simulink model "all_phase"  (Simulink 10.0)
settings: Solver=ode45  StartTime=0.0  StopTime=10.0  RelTol=1e-3  EnableMultiTasking=on
settings Model: Creator=bhisma  LastModifiedBy=bhisma
settings DataIOCC: LimitDataPoints=on  SignalLoggingSaveFormat=ModelDataLogs  SignalLoggingName=sigsOut
settings OptimizationCC: BlockReduction=off  BooleanDataType=off  LifeSpan=auto
settings DebuggingCC: SaveWithParameterizedLinksMsg=none  SignalResolutionControl=TryResolveAllWithWarning  MultiTaskDSMMsg=warning  MultiTaskCondExecSysMsg=none  SFUnexpectedBacktrackingDiag=error  SFNoUnconditionalDefaultTransitionDiag=error  SFExecutionAtInitializationDiag=warning  ArithmeticOperatorsInVariantConditions=error
settings HardwareCC: TargetUnknown=on
settings SFSimCC: SimUseLocalCustomCode=on  CustomCodeUndefinedFunction=FilterOut
settings RTWCC: RTWUseLocalCustomCode=on
settings CodeAppCC: StateflowObjectComments=off
settings GRTTargetCC: TargetLangStandard=C99 (ISO)

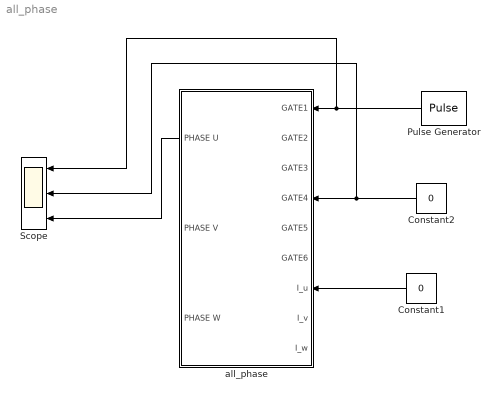
== system all_phase ==
  Constant1 : Constant  Value=0
  Constant2 : Constant  Value=0
  Pulse Generator : DiscretePulseGenerator  PulseType=Time based  Amplitude=100  Period=0.2  PulseWidth=50
  Scope : Scope  NumInputPorts=3
  all_phase : Subsystem  mask{BV=160}
      mask prompts: BV "Battery voltage for excitation"
      mask help: This is an inverter. Double click the block to enter the battery voltage
  wires:
  Pulse Generator/1 -> all_phase/1(GATE1), Scope/1
  Constant2/1 -> all_phase/4(GATE4), Scope/2
  Constant1/1 -> all_phase/7(I_u)
  all_phase/1(PHASE U) -> Scope/3

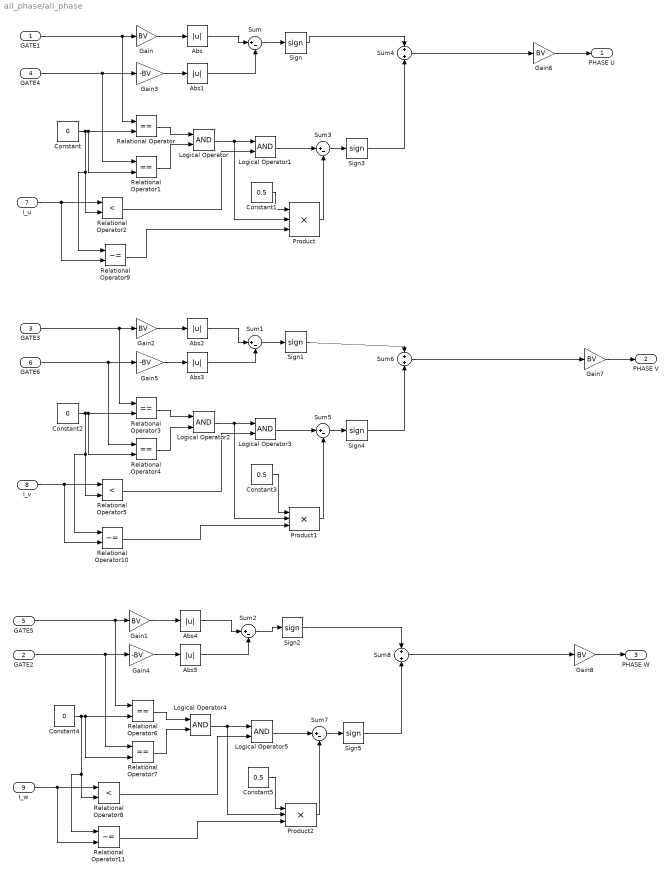
== system all_phase/all_phase ==
  GATE1 : Inport
  GATE2 : Inport  Port=2
  GATE3 : Inport  Port=3
  GATE4 : Inport  Port=4
  GATE5 : Inport  Port=5
  GATE6 : Inport  Port=6
  I_u : Inport  Port=7
  I_v : Inport  Port=8
  I_w : Inport  Port=9
  Abs{,1..5} (6 alike) : Abs  SaturateOnIntegerOverflow=on
  Constant : Constant  Value=0
  Constant1 : Constant  Value=0.5
  Constant2 : Constant  Value=0
  Constant3 : Constant  Value=0.5
  Constant4 : Constant  Value=0
  Constant5 : Constant  Value=0.5
  Gain{,1..2,6..8} (6 alike) : Gain  Gain=BV  SaturateOnIntegerOverflow=on  OutDataTypeStr=Inherit: Same as input  ParamDataTypeStr=Inherit: Same as input
  Gain3 : Gain  Gain=-BV  SaturateOnIntegerOverflow=on  OutDataTypeStr=Inherit: Same as input  ParamDataTypeStr=Inherit: Same as input
  Gain4 : Gain  Gain=-BV  SaturateOnIntegerOverflow=on  OutDataTypeStr=Inherit: Same as input  ParamDataTypeStr=Inherit: Same as input
  Gain5 : Gain  Gain=-BV  SaturateOnIntegerOverflow=on  OutDataTypeStr=Inherit: Same as input  ParamDataTypeStr=Inherit: Same as input
  Logical Operator{,1..5} (6 alike) : Logic  AllPortsSameDT=off
  Product : Product  Inputs=3  SaturateOnIntegerOverflow=on  OutDataTypeStr=Inherit: Same as first input
  Product1 : Product  Inputs=3  SaturateOnIntegerOverflow=on  OutDataTypeStr=Inherit: Same as first input
  Product2 : Product  Inputs=3  SaturateOnIntegerOverflow=on  OutDataTypeStr=Inherit: Same as first input
  Relational Operator{,1,3..4,6..7} (6 alike) : RelationalOperator  Operator===  RndMeth=Nearest
  Relational Operator10 : RelationalOperator  Operator=~=  RndMeth=Nearest
  Relational Operator11 : RelationalOperator  Operator=~=  RndMeth=Nearest
  Relational Operator2 : RelationalOperator  Operator=<  RndMeth=Nearest
  Relational Operator5 : RelationalOperator  Operator=<  RndMeth=Nearest
  Relational Operator8 : RelationalOperator  Operator=<  RndMeth=Nearest
  Relational Operator9 : RelationalOperator  Operator=~=  RndMeth=Nearest
  Sign{,1..5} (6 alike) : Signum
  Sum{,1..3,5,7} (6 alike) : Sum  Inputs=|+-  SaturateOnIntegerOverflow=on  InputSameDT=on  OutDataTypeStr=Inherit: Same as first input
  Sum4 : Sum  SaturateOnIntegerOverflow=on  InputSameDT=on  OutDataTypeStr=Inherit: Same as first input
  Sum6 : Sum  SaturateOnIntegerOverflow=on  InputSameDT=on  OutDataTypeStr=Inherit: Same as first input
  Sum8 : Sum  SaturateOnIntegerOverflow=on  InputSameDT=on  OutDataTypeStr=Inherit: Same as first input
  PHASE U : Outport
  PHASE V : Outport  Port=2
  PHASE W : Outport  Port=3
  wires:
  GATE1/1 -> Gain/1, Relational Operator/1
  GATE5/1 -> Gain1/1, Relational Operator6/1
  GATE3/1 -> Gain2/1, Relational Operator3/1
  GATE4/1 -> Gain3/1, Relational Operator1/1
  GATE2/1 -> Gain4/1, Relational Operator7/1
  GATE6/1 -> Gain5/1, Relational Operator4/1
  Gain/1 -> Abs/1
  Gain3/1 -> Abs1/1
  Gain2/1 -> Abs2/1
  Gain5/1 -> Abs3/1
  Gain1/1 -> Abs4/1
  Gain4/1 -> Abs5/1
  Abs/1 -> Sum/1
  Abs1/1 -> Sum/2
  Abs2/1 -> Sum1/1
  Abs3/1 -> Sum1/2
  Abs4/1 -> Sum2/1
  Abs5/1 -> Sum2/2
  Sum/1 -> Sign/1
  Sum1/1 -> Sign1/1
  Sum2/1 -> Sign2/1
  Gain8/1 -> PHASE W/1
  Gain7/1 -> PHASE V/1
  Gain6/1 -> PHASE U/1
  Constant/1 -> Relational Operator/2, Relational Operator1/2, Relational Operator2/2, Relational Operator9/1
  Relational Operator/1 -> Logical Operator/1
  Relational Operator1/1 -> Logical Operator/2
  I_u/1 -> Relational Operator2/1, Relational Operator9/2
  Logical Operator/1 -> Logical Operator1/1, Product/2
  Relational Operator2/1 -> Logical Operator1/2
  Logical Operator1/1 -> Sum3/1
  Sum3/1 -> Sign3/1
  Sign/1 -> Sum4/1
  Sign3/1 -> Sum4/2
  Sum4/1 -> Gain6/1
  Constant2/1 -> Relational Operator4/2, Relational Operator3/2, Relational Operator5/2, Relational Operator10/1
  Relational Operator3/1 -> Logical Operator2/1
  Relational Operator4/1 -> Logical Operator2/2
  I_v/1 -> Relational Operator5/1, Relational Operator10/2
  Logical Operator2/1 -> Logical Operator3/1, Product1/2
  Relational Operator5/1 -> Logical Operator3/2
  Logical Operator3/1 -> Sum5/1
  Sum5/1 -> Sign4/1
  Sign1/1 -> Sum6/1
  Sign4/1 -> Sum6/2
  Sum6/1 -> Gain7/1
  Constant4/1 -> Relational Operator6/2, Relational Operator7/2, Relational Operator8/2, Relational Operator11/1
  Relational Operator6/1 -> Logical Operator4/1
  Relational Operator7/1 -> Logical Operator4/2
  I_w/1 -> Relational Operator8/1, Relational Operator11/2
  Logical Operator4/1 -> Logical Operator5/1, Product2/2
  Relational Operator8/1 -> Logical Operator5/2
  Logical Operator5/1 -> Sum7/1
  Sum7/1 -> Sign5/1
  Sign5/1 -> Sum8/2
  Sign2/1 -> Sum8/1
  Sum8/1 -> Gain8/1
  Constant1/1 -> Product/1
  Product/1 -> Sum3/2
  Constant3/1 -> Product1/1
  Product1/1 -> Sum5/2
  Constant5/1 -> Product2/1
  Product2/1 -> Sum7/2
  Relational Operator9/1 -> Product/3
  Relational Operator10/1 -> Product1/3
  Relational Operator11/1 -> Product2/3
